simulink model "test_co_sim_redis"  (R2024a)
settings: Solver=FixedStepDiscrete  StartTime=0.0  StopTime=10.0  FixedStep=1e-3  RelTol=1e-3
values from neighbouring files (symbols this model uses):
  Kd_IPF = [0 0 0 0 0 0 0 0 0 0 0 0]    [load_data.m]
  Ki_IPF = [0 0 0 0 0 0 0 0 0 0 0 0]    [load_data.m]
  Kp_IPF = [2 2 2 2 2 2 2 2 2 2 2 2]    [load_data.m]
  Maa = [0.7635    0.2320    0.0658    0.0074    0.0039    0.1363    0.0434    0.0473    0.0270    0.0150    0.0108   -0.0017 ... (first row only)    [load_data.m]
  Ra = [0         0         0         0         0         0         0         0         0         0         0         0 ... (first row only)    [load_data.m]
  T_IPF = diag([1 1 1 1 1 1 1 1 1 1 1 0].')    [load_data.m]
libraries: slpidlib x1
settings Model: Creator=ravenst1  LastModifiedBy=deshazere
settings SolverCC: AlgebraicLoopSolver=TrustRegion
settings DebuggingCC: UnconnectedInputMsg=warning  UnconnectedOutputMsg=warning  UnconnectedLineMsg=warning
settings ModelReferenceCC: EnableRefExpFcnMdlSchedulingChecks=on
settings RTWCC: GPUComputeCapability=3.5  DLArmComputeVersion=19.05

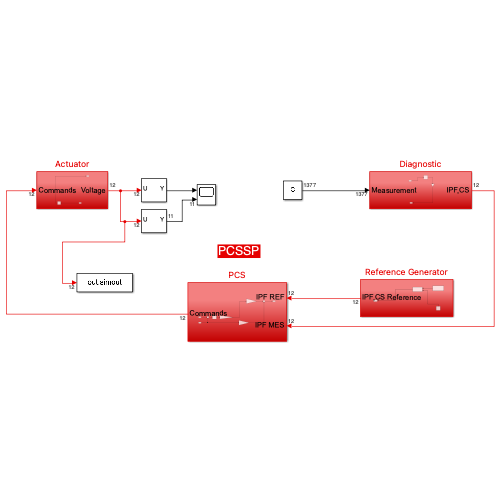
[thumbnail: Simulink's stored preview of the top-level diagram]
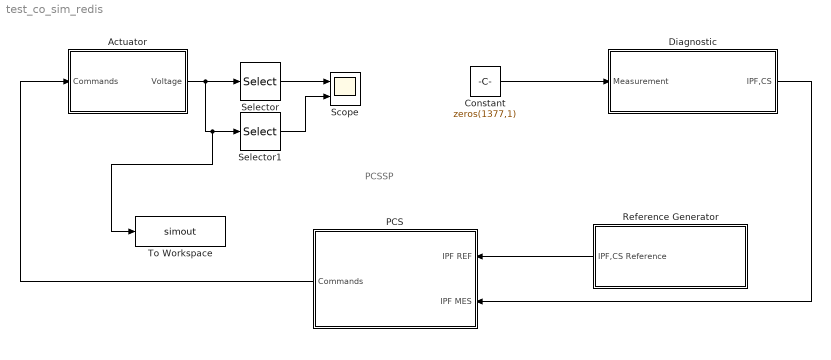
== system test_co_sim_redis ==
  note: PCSSP
  Actuator : Subsystem
  Constant : Constant  Value=zeros(1377,1)
  Diagnostic : Subsystem
  PCS : Subsystem
  Reference Generator : Subsystem
  Scope : Scope  NumInputPorts=2
  Selector : Selector  IndexOptions=Index vector (dialog)  Indices=1  OutputSizes=1
  Selector1 : Selector  IndexOptions=Index vector (dialog)  Indices=[2:12]  OutputSizes=1
  To Workspace : ToWorkspace  VariableName=simout  SaveFormat=Timeseries  SampleTime=-1
  wires:
  PCS/1(Commands) -> Actuator/1(Commands)
  Constant/1 -> Diagnostic/1(Measurement)
  Diagnostic/1(IPF,CS) -> PCS/2(IPF MES)
  Reference Generator/1(IPF,CS Reference) -> PCS/1(IPF REF)
  Selector/1 -> Scope/1
  Actuator/1(Voltage) -> To Workspace/1, Selector1/1, Selector/1
  Selector1/1 -> Scope/2

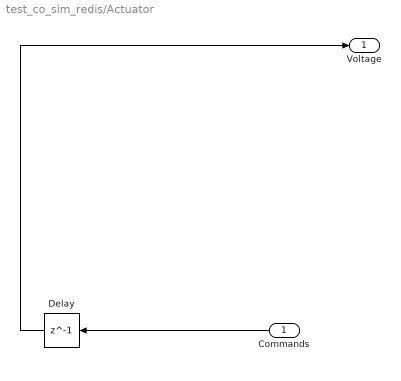
== system test_co_sim_redis/Actuator ==
  Commands : Inport
  Delay : Delay  DelayLength=1
  Voltage : Outport
  wires:
  Commands/1 -> Delay/1
  Delay/1 -> Voltage/1

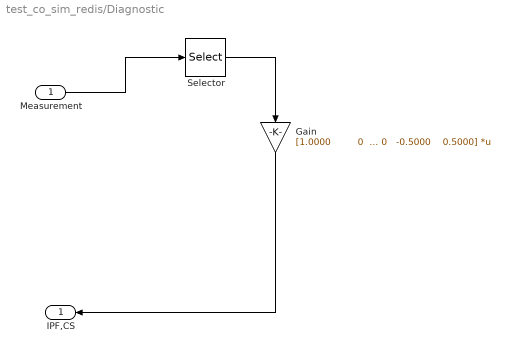
== system test_co_sim_redis/Diagnostic ==
  Measurement : Inport
  Gain : Gain  Gain=|  Multiplication=Matrix(K*u)
      | [1.0000         0         0         0         0         0         0         0         0         0         0         0         0         0
      |          0    1.0000         0         0         0         0         0         0         0         0         0         0         0         0
      |          0         0    0.5000    0.5000         0         0         0         0         0         0         0         0         0         0
      |          0         0         0         0    1.0000         0         0         0         0         0         0         0         0         0
      |          0         0         0         0         0    1.0000         0         0         0         0         0         0         0         0
      |          0         0         0         0         0         0    1.0000         0         0         0         0         0         0         0
      |          0         0         0         0         0         0         0    1.0000         0         0         0         0         0         0
      |          0         0         0         0         0         0         0         0    1.0000         0         0         0         0         0
      |          0         0         0         0         0         0         0         0         0    1.0000         0         0         0         0
      |          0         0         0         0         0         0         0         0         0         0    1.0000         0         0         0
      |          0         0         0         0         0         0         0         0         0         0         0    1.0000         0         0
      |          0         0         0         0         0         0         0         0         0         0         0         0   -0.5000    0.5000]
  Selector : Selector  IndexOptions=Index vector (dialog)  Indices=[iter_system.output_map.cc.start:iter_system.output_map.cc.end]  OutputSizes=1
  IPF,CS : Outport
  wires:
  Selector/1 -> Gain/1
  Measurement/1 -> Selector/1
  Gain/1 -> IPF,CS/1

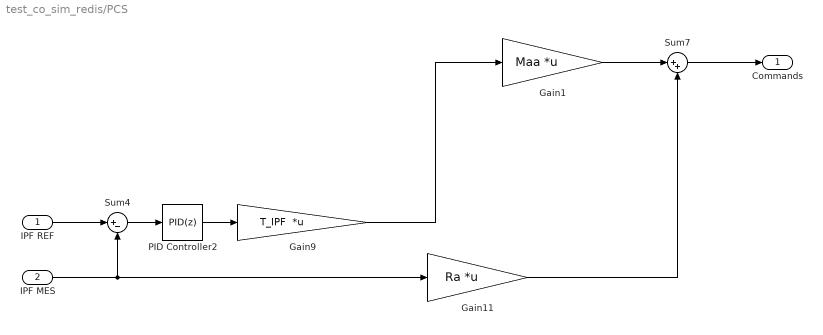
== system test_co_sim_redis/PCS ==
  IPF REF : Inport
  IPF MES : Inport  Port=2
  Gain1 : Gain  Gain=Maa  Multiplication=Matrix(K*u)
  Gain11 : Gain  Gain=Ra  Multiplication=Matrix(K*u)
  Gain9 : Gain  Gain=T_IPF  Multiplication=Matrix(K*u)
  PID Controller2 : slpidlib/PID Controller  Controller=PID  Form=Parallel  TimeDomain=Discrete-time  UseExternalTs=off  SampleTime=-1  IntegratorMethod=Forward Euler  FilterMethod=Forward Euler  ControllerParametersSource=internal  P=Kp_IPF  I=Ki_IPF  UseKiTs=off  D=Kd_IPF  UseExternalDerivativeSource=off  N=100  UseFilter=on  TunerSelectOption=Transfer Function Based (PID Tuner App)  InitialConditionSource=internal  InitialConditionForIntegrator=0  InitialConditionForFilter=0  DifferentiatorICPrevScaledInput=0  ExternalReset=none  TrackingMode=off  Kt=1  LimitOutput=off  SatLimitsSource=internal  UpperSaturationLimit=inf  LowerSaturationLimit=-inf  LinearizeAsGain=on  AntiWindupMode=none  Kb=1  LimitIntegrator=off  UpperIntegratorSaturationLimit=inf  LowerIntegratorSaturationLimit=-inf  POutMin=[]  POutMax=[]  IOutMin=[]  IOutMax=[]  DOutMin=[]  DOutMax=[]  NOutMin=[]  NOutMax=[]  SumOutMin=[]  SumOutMax=[]  SaturationOutMin=[]  SaturationOutMax=[]  PParamMin=[]  PParamMax=[]  IParamMin=[]  IParamMax=[]  DParamMin=[]  DParamMax=[]  NParamMin=[]  NParamMax=[]  KbParamMin=[]  KbParamMax=[]  KtParamMin=[]  KtParamMax=[]  KbOutMin=[]  KbOutMax=[]  KtOutMin=[]  KtOutMax=[]  IntegratorOutMin=[]  IntegratorOutMax=[]  FilterOutMin=[]  FilterOutMax=[]  SumI1OutMin=[]  SumI1OutMax=[]  SumI2OutMin=[]  SumI2OutMax=[]  SumI3OutMin=[]  SumI3OutMax=[]  SumI4OutMin=[]  SumI4OutMax=[]  SumDOutMin=[]  SumDOutMax=[]  DifferentiatorOutMin=[]  DifferentiatorOutMax=[]  FilterDiffOutCoefMin=[]  FilterDiffOutCoefMax=[]  ReciprocalOutMin=[]  ReciprocalOutMax=[]  SumDenOutMin=[]  SumDenOutMax=[]  SumNumOutMin=[]  SumNumOutMax=[]  DivideOutMin=[]  DivideOutMax=[]  UdiffTsProdOutMin=[]  UdiffTsProdOutMax=[]  NTsProdOutMin=[]  NTsProdOutMax=[]  UintegralTsProdOutMin=[]  UintegralTsProdOutMax=[]  UngainTsProdOutMin=[]  UngainTsProdOutMax=[]  ClampingZeroOutDataTypeStr=Inherit: Inherit via back propagation  ClampingZeroOutMin=[]  ClampingZeroOutMax=[]  FilterDenConstantOutDataTypeStr=Inherit: Inherit via back propagation  FilterDenConstantOutMin=[]  FilterDenConstantOutMax=[]  PCopyOutDataTypeStr=Inherit: Inherit via back propagation  PCopyOutMin=[]  PCopyOutMax=[]  NCopyOutDataTypeStr=Inherit: Inherit via back propagation  NCopyOutMin=[]  NCopyOutMax=[]  IntegratorContinuousStateAttributes=''  IntegratorStateMustResolveToSignalObject=off  IntegratorRTWStateStorageClass=Auto  FilterContinuousStateAttributes=''  FilterStateMustResolveToSignalObject=off  FilterRTWStateStorageClass=Auto  ParallelPVariant=InternalParameters  IdealPVariant=Disabled  IVariant=InternalParameters  DVariant=InternalParameters  IntegratorVariant=Discrete  SatVariant=Disabled  AWVariant=Passthrough  PCopyVariant=Disabled  TRVariant=Disabled  FdbkBlocksVariant=Forward  IdealPFdbkVariant=Disabled  SatFdbkVariant=Disabled  DerivativeFilterVariant=ForwardEulerFilter  NVariant=InternalParameters  NCopyVariant=Disabled  FilterICVariant=InternalICsFilter  IntegratorICVariant=InternalICs  ExternalResetVariant=Disabled  TRSumVariant=Passthrough  SumFdbkVariant=Disabled  SumVariant=Sum_PID  TsampFilterVariant=InternalTs  TsampNgainVariant=Passthrough  TsampIntegralVariant=Disabled_SignalSpec  ExternalSaturationOutDataTypeStr=Inherit: Same as second input  DerivativeSourceVariant=ErrorSignal
  Sum4 : Sum  Inputs=|+-
  Sum7 : Sum  Inputs=|++
  Commands : Outport
  wires:
  Sum4/1 -> PID Controller2/1
  IPF REF/1 -> Sum4/1
  Gain9/1 -> Gain1/1
  Gain11/1 -> Sum7/2
  Gain1/1 -> Sum7/1
  Sum7/1 -> Commands/1
  IPF MES/1 -> Gain11/1, Sum4/2
  PID Controller2/1 -> Gain9/1

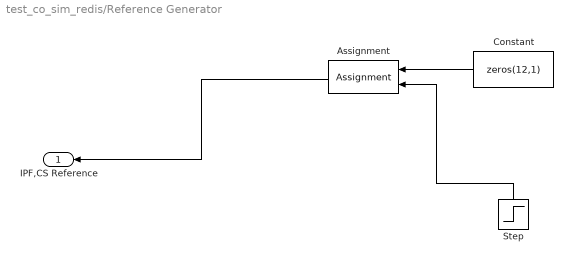
== system test_co_sim_redis/Reference Generator ==
  Assignment : Assignment  DiagnosticForDimensions=Warning  IndexOptions=Index vector (dialog)  Indices=3  OutputSizes=1
  Constant : Constant  Value=zeros(12,1)
  Step : Step  After=1e3  SampleTime=0
  IPF,CS Reference : Outport
  wires:
  Constant/1 -> Assignment/1
  Step/1 -> Assignment/2
  Assignment/1 -> IPF,CS Reference/1
